simulink model "TypeA_siso180515_export"  (R2016a)
settings: Solver=ode45  StartTime=0.0  StopTime=12.0  RelTol=1e-3
values from neighbouring files (symbols this model uses):
  gain_actIML = 2.1e-7*1.e+6*20/(2^16)/magIM(inddc)*gain_actIML    [TypeA_reconstruction.m]
  gain_actMNL = 5.1e-6*1.e+6*20/(2^16)/magMN(inddc)*gain_actMNL    [TypeA_reconstruction.m]
  gain_actTML = 1.7e-7*1.e+6*20/(2^16)/magTM(inddc)*gain_actTML    [TypeA_reconstruction.m]
  gainBFL = 0    [main.m]
  gainIPL = 0    [main.m]
  sys1 = sys1_exp    [check_exportvsmake.m]    (also in sumcon2mdlconst_typeA.m = sus.ss)
undefined symbols (not defined in the file or in its folder): cMat_BF, cMat_IM, cMat_MN, cMat_TM, gain_actBFGAS, gain_actBFL, gain_actBFP, gain_actBFR, gain_actBFT, gain_actBFV, gain_actBFY, gain_actF0GAS, gain_actF1GAS, gain_actF2GAS, gain_actF3GAS, gain_actIMP, gain_actIMR, gain_actIMT, gain_actIMV, gain_actIMY, gain_actIPL, gain_actIPT, gain_actIPY, gain_actMNP, gain_actMNR, gain_actMNT, gain_actMNV, gain_actMNY, gain_actTMP, gain_actTMY, gainBFGAS, gainBFP, gainBFR, gainBFT, gainBFV, gainBFY, gainF0GAS, gainF1GAS, gainF2GAS, gainF3GAS, gainHieBFP, gainHieBFR, gainHieBFY, gainHieIML, gainHieIMP, gainHieIMY, gainHieIPL, gainHieIPY, gainHieMNL, gainHieMNP, gainHieMNY, gainIML, gainIMP, gainIMR, gainIMT, gainIMV, gainIMY, gainIPT, gainIPY, gainISC_TML ... (+18)
libraries: cstblocks x57
(part 2 of 2)

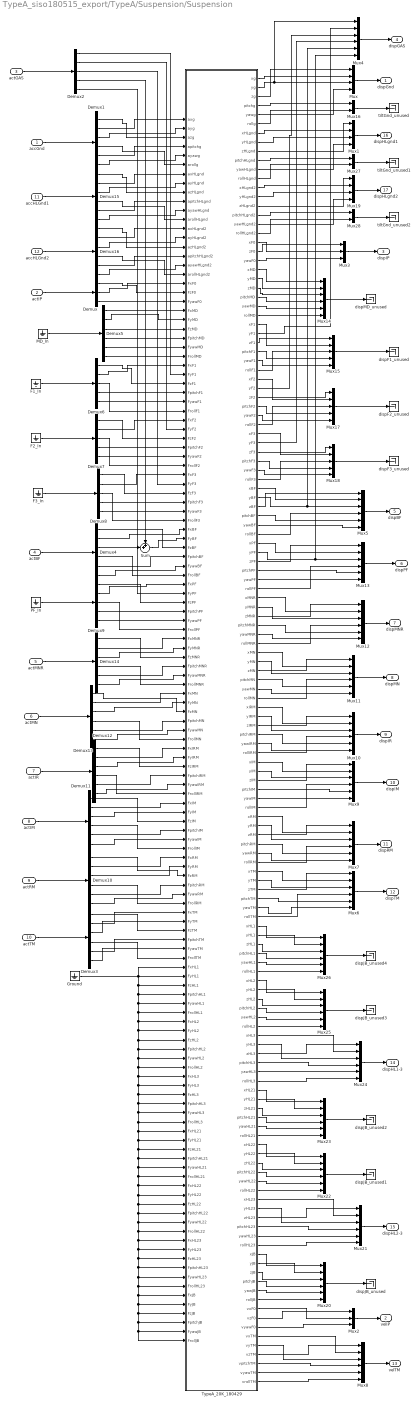
== system TypeA_siso180515_export/TypeA/Suspension/Suspension ==
  accGnd : Inport
  actIP : Inport  Port=2
  actGAS : Inport  Port=3
  actBF : Inport  Port=4
  actMNR : Inport  Port=5
  actMN : Inport  Port=6
  actIR : Inport  Port=7
  actIM : Inport  Port=8
  actRM : Inport  Port=9
  actTM : Inport  Port=10
  accHLGnd1 : Inport  Port=11
  accHLGnd2 : Inport  Port=12
  Demux : Demux  Outputs=3
  Demux{1,3..5,10..16} (11 alike) : Demux  Outputs=6
  Demux{2,6..9} (5 alike) : Demux  Outputs=5
  F1_In : Ground
  F2_In : Ground
  F3_In : Ground
  Ground : Ground
  MD_In : Ground
  Mux : Mux
  Mux1 : Mux
  Mux{4..14,20..26} (18 alike) : Mux  Inputs=6
  Mux15 : Mux  Inputs=5
  Mux16 : Mux  Inputs=2
  Mux17 : Mux  Inputs=5
  Mux18 : Mux  Inputs=5
  Mux19 : Mux
  Mux2 : Mux  Inputs=3
  Mux27 : Mux  Inputs=2
  Mux28 : Mux  Inputs=2
  Mux3 : Mux  Inputs=3
  PF_In : Ground
  Sum : Sum  Inputs=++|
  TypeA_20K_180429 : Subsystem
  dispF1_unused : Terminator
  dispF2_unused : Terminator
  dispF3_unused : Terminator
  dispJB_unused{,1..4} (5 alike) : Terminator
  dispMD_unused : Terminator
  tiltGnd_unused : Terminator
  tiltGnd_unused1 : Terminator
  tiltGnd_unused2 : Terminator
  dispGnd : Outport
  velIP : Outport  Port=2
  dispIP : Outport  Port=3
  dispGAS : Outport  Port=4
  dispBF : Outport  Port=5
  dispPF : Outport  Port=6
  dispMNR : Outport  Port=7
  dispMN : Outport  Port=8
  dispIR : Outport  Port=9
  dispIM : Outport  Port=10
  dispRM : Outport  Port=11
  dispTM : Outport  Port=12
  velTM : Outport  Port=13
  dispHL1-3 : Outport  Port=14
  dispHL2-3 : Outport  Port=15
  dispHLgnd1 : Outport  Port=16
  dispHLgnd2 : Outport  Port=17
  wires:
  Mux/1 -> dispGnd/1
  Mux2/1 -> velIP/1
  Mux3/1 -> dispIP/1
  Mux4/1 -> dispGAS/1
  Mux5/1 -> dispBF/1
  Mux6/1 -> dispTM/1
  actIP/1 -> Demux/1
  accGnd/1 -> Demux1/1
  actTM/1 -> Demux3/1
  Demux4/3 -> Sum/2
  Demux2/4 -> Sum/1
  Demux2/5 -> TypeA_20K_180429/53(FyPF)
  actBF/1 -> Demux4/1
  actGAS/1 -> Demux2/1
  MD_In/1 -> Demux5/1
  Demux5/1 -> TypeA_20K_180429/22(FxMD)
  Demux5/2 -> TypeA_20K_180429/23(FyMD)
  Demux5/3 -> TypeA_20K_180429/24(FzMD)
  Demux5/4 -> TypeA_20K_180429/25(FpitchMD)
  Demux5/5 -> TypeA_20K_180429/26(FyawMD)
  Demux5/6 -> TypeA_20K_180429/27(FrollMD)
  Demux2/1 -> TypeA_20K_180429/29(FyF1)
  Demux2/2 -> TypeA_20K_180429/35(FyF2)
  Demux2/3 -> TypeA_20K_180429/41(FyF3)
  F1_In/1 -> Demux6/1
  F2_In/1 -> Demux7/1
  F3_In/1 -> Demux8/1
  Demux4/1 -> TypeA_20K_180429/48(FzBF)
  PF_In/1 -> Demux9/1
  actRM/1 -> Demux10/1
  actIM/1 -> Demux11/1
  actIR/1 -> Demux12/1
  actMN/1 -> Demux13/1
  actMNR/1 -> Demux14/1
  Demux10/5 -> TypeA_20K_180429/85(FpitchRM)
  Demux10/4 -> TypeA_20K_180429/87(FrollRM)
  Demux10/3 -> TypeA_20K_180429/83(FyRM)
  Demux10/1 -> TypeA_20K_180429/84(FzRM)
  Demux10/2 -> TypeA_20K_180429/82(FxRM)
  Demux3/3 -> TypeA_20K_180429/89(FyTM)
  Demux3/1 -> TypeA_20K_180429/90(FzTM)
  Demux3/2 -> TypeA_20K_180429/88(FxTM)
  Demux3/4 -> TypeA_20K_180429/93(FrollTM)
  Demux3/5 -> TypeA_20K_180429/91(FpitchTM)
  Demux3/6 -> TypeA_20K_180429/92(FyawTM)
  Mux7/1 -> dispRM/1
  Mux8/1 -> velTM/1
  Mux9/1 -> dispIM/1
  Mux10/1 -> dispIR/1
  Mux11/1 -> dispMN/1
  Mux12/1 -> dispMNR/1
  Mux13/1 -> dispPF/1
  Mux14/1 -> dispMD_unused/1
  Mux15/1 -> dispF1_unused/1
  Mux16/1 -> tiltGnd_unused/1
  Mux17/1 -> dispF2_unused/1
  Mux18/1 -> dispF3_unused/1
  TypeA_20K_180429/1(xg) -> Mux/2
  TypeA_20K_180429/3(zg) -> Mux/1
  TypeA_20K_180429/138(vyawF0) -> Mux2/3
  TypeA_20K_180429/19(xF0) -> Mux3/2
  TypeA_20K_180429/20(zF0) -> Mux3/1
  TypeA_20K_180429/21(yawF0) -> Mux3/3
  TypeA_20K_180429/24(zMD) -> Mux14/3
  TypeA_20K_180429/25(pitchMD) -> Mux14/4
  TypeA_20K_180429/26(yawMD) -> Mux14/5
  TypeA_20K_180429/27(rollMD) -> Mux14/6
  TypeA_20K_180429/29(yF1) -> Mux4/2
  TypeA_20K_180429/35(yF2) -> Mux4/3
  TypeA_20K_180429/41(yF3) -> Mux4/4
  TypeA_20K_180429/47(yBF) -> Mux5/3, Mux4/5
  TypeA_20K_180429/53(yPF) -> Mux13/3, Mux4/6
  TypeA_20K_180429/30(zF1) -> Mux15/1
  TypeA_20K_180429/28(xF1) -> Mux15/2
  TypeA_20K_180429/32(yawF1) -> Mux15/5
  TypeA_20K_180429/33(rollF1) -> Mux15/3
  TypeA_20K_180429/31(pitchF1) -> Mux15/4
  TypeA_20K_180429/36(zF2) -> Mux17/1
  TypeA_20K_180429/34(xF2) -> Mux17/2
  TypeA_20K_180429/39(rollF2) -> Mux17/3
  TypeA_20K_180429/38(yawF2) -> Mux17/5
  TypeA_20K_180429/37(pitchF2) -> Mux17/4
  TypeA_20K_180429/42(zF3) -> Mux18/1
  TypeA_20K_180429/40(xF3) -> Mux18/2
  TypeA_20K_180429/44(yawF3) -> Mux18/5
  TypeA_20K_180429/43(pitchF3) -> Mux18/4
  TypeA_20K_180429/45(rollF3) -> Mux18/3
  TypeA_20K_180429/49(pitchBF) -> Mux5/5
  TypeA_20K_180429/50(yawBF) -> Mux5/6
  TypeA_20K_180429/51(rollBF) -> Mux5/4
  TypeA_20K_180429/46(xBF) -> Mux5/2
  TypeA_20K_180429/48(zBF) -> Mux5/1
  TypeA_20K_180429/56(yawPF) -> Mux13/6
  TypeA_20K_180429/54(zPF) -> Mux13/1
  TypeA_20K_180429/52(xPF) -> Mux13/2
  TypeA_20K_180429/57(rollPF) -> Mux13/4
  TypeA_20K_180429/55(pitchPF) -> Mux13/5
  TypeA_20K_180429/58(xMNR) -> Mux12/2
  TypeA_20K_180429/62(yawMNR) -> Mux12/6
  TypeA_20K_180429/59(yMNR) -> Mux12/3
  TypeA_20K_180429/63(rollMNR) -> Mux12/4
  TypeA_20K_180429/60(zMNR) -> Mux12/1
  TypeA_20K_180429/61(pitchMNR) -> Mux12/5
  TypeA_20K_180429/69(rollMN) -> Mux11/4
  TypeA_20K_180429/66(zMN) -> Mux11/1
  TypeA_20K_180429/65(yMN) -> Mux11/3
  TypeA_20K_180429/64(xMN) -> Mux11/2
  TypeA_20K_180429/68(yawMN) -> Mux11/6
  TypeA_20K_180429/67(pitchMN) -> Mux11/5
  TypeA_20K_180429/73(pitchIRM) -> Mux10/5
  TypeA_20K_180429/71(yIRM) -> Mux10/3
  TypeA_20K_180429/74(yawIRM) -> Mux10/6
  TypeA_20K_180429/75(rollIRM) -> Mux10/4
  TypeA_20K_180429/70(xIRM) -> Mux10/2
  TypeA_20K_180429/72(zIRM) -> Mux10/1
  TypeA_20K_180429/78(zIM) -> Mux9/1
  TypeA_20K_180429/77(yIM) -> Mux9/3
  TypeA_20K_180429/76(xIM) -> Mux9/2
  TypeA_20K_180429/141(vzTM) -> Mux8/1
  TypeA_20K_180429/139(vxTM) -> Mux8/2
  TypeA_20K_180429/140(vyTM) -> Mux8/3
  TypeA_20K_180429/142(vpitchTM) -> Mux8/4
  TypeA_20K_180429/143(vyawTM) -> Mux8/5
  TypeA_20K_180429/144(vrollTM) -> Mux8/6
  TypeA_20K_180429/90(zTM) -> Mux6/1
  TypeA_20K_180429/88(xTM) -> Mux6/2
  TypeA_20K_180429/89(yTM) -> Mux6/3
  TypeA_20K_180429/84(zRM) -> Mux7/1
  TypeA_20K_180429/82(xRM) -> Mux7/2
  TypeA_20K_180429/83(yRM) -> Mux7/3
  TypeA_20K_180429/81(rollIM) -> Mux9/4
  TypeA_20K_180429/79(pitchIM) -> Mux9/5
  TypeA_20K_180429/80(yawIM) -> Mux9/6
  TypeA_20K_180429/87(rollRM) -> Mux7/4
  TypeA_20K_180429/85(pitchRM) -> Mux7/5
  TypeA_20K_180429/86(yawRM) -> Mux7/6
  TypeA_20K_180429/93(rollTM) -> Mux6/4
  TypeA_20K_180429/91(pitchTM) -> Mux6/5
  TypeA_20K_180429/92(yawTM) -> Mux6/6
  TypeA_20K_180429/22(xMD) -> Mux14/1
  TypeA_20K_180429/23(yMD) -> Mux14/2
  TypeA_20K_180429/136(vxF0) -> Mux2/2
  TypeA_20K_180429/137(vzF0) -> Mux2/1
  TypeA_20K_180429/2(yg) -> Mux4/1, Mux/3
  TypeA_20K_180429/5(yawg) -> Mux/4
  TypeA_20K_180429/4(pitchg) -> Mux16/1
  TypeA_20K_180429/6(rollg) -> Mux16/2
  Demux10/6 -> TypeA_20K_180429/86(FyawRM)
  Demux11/1 -> TypeA_20K_180429/78(FzIM)
  Demux11/2 -> TypeA_20K_180429/76(FxIM)
  Demux11/3 -> TypeA_20K_180429/77(FyIM)
  Demux11/4 -> TypeA_20K_180429/81(FrollIM)
  Demux11/5 -> TypeA_20K_180429/79(FpitchIM)
  Demux11/6 -> TypeA_20K_180429/80(FyawIM)
  Demux12/1 -> TypeA_20K_180429/72(FzIRM)
  Demux12/2 -> TypeA_20K_180429/70(FxIRM)
  Demux12/3 -> TypeA_20K_180429/71(FyIRM)
  Demux12/4 -> TypeA_20K_180429/75(FrollIRM)
  Demux12/5 -> TypeA_20K_180429/73(FpitchIRM)
  Demux12/6 -> TypeA_20K_180429/74(FyawIRM)
  Demux13/1 -> TypeA_20K_180429/66(FzMN)
  Demux13/2 -> TypeA_20K_180429/64(FxMN)
  Demux13/3 -> TypeA_20K_180429/65(FyMN)
  Demux13/4 -> TypeA_20K_180429/69(FrollMN)
  Demux13/5 -> TypeA_20K_180429/67(FpitchMN)
  Demux13/6 -> TypeA_20K_180429/68(FyawMN)
  Demux14/1 -> TypeA_20K_180429/60(FzMNR)
  Demux14/2 -> TypeA_20K_180429/58(FxMNR)
  Demux14/3 -> TypeA_20K_180429/59(FyMNR)
  Demux14/4 -> TypeA_20K_180429/63(FrollMNR)
  Demux14/5 -> TypeA_20K_180429/61(FpitchMNR)
  Demux14/6 -> TypeA_20K_180429/62(FyawMNR)
  Demux9/1 -> TypeA_20K_180429/54(FzPF)
  Demux9/2 -> TypeA_20K_180429/52(FxPF)
  Demux9/3 -> TypeA_20K_180429/57(FrollPF)
  Demux9/4 -> TypeA_20K_180429/55(FpitchPF)
  Demux9/5 -> TypeA_20K_180429/56(FyawPF)
  Demux4/2 -> TypeA_20K_180429/46(FxBF)
  Sum/1 -> TypeA_20K_180429/47(FyBF)
  Demux4/4 -> TypeA_20K_180429/51(FrollBF)
  Demux4/5 -> TypeA_20K_180429/49(FpitchBF)
  Demux4/6 -> TypeA_20K_180429/50(FyawBF)
  Demux8/1 -> TypeA_20K_180429/42(FzF3)
  Demux8/2 -> TypeA_20K_180429/40(FxF3)
  Demux8/3 -> TypeA_20K_180429/45(FrollF3)
  Demux8/4 -> TypeA_20K_180429/43(FpitchF3)
  Demux8/5 -> TypeA_20K_180429/44(FyawF3)
  Demux7/1 -> TypeA_20K_180429/36(FzF2)
  Demux7/2 -> TypeA_20K_180429/34(FxF2)
  Demux7/3 -> TypeA_20K_180429/39(FrollF2)
  Demux7/4 -> TypeA_20K_180429/37(FpitchF2)
  Demux7/5 -> TypeA_20K_180429/38(FyawF2)
  Demux6/1 -> TypeA_20K_180429/30(FzF1)
  Demux6/2 -> TypeA_20K_180429/28(FxF1)
  Demux6/3 -> TypeA_20K_180429/33(FrollF1)
  Demux6/4 -> TypeA_20K_180429/31(FpitchF1)
  Demux6/5 -> TypeA_20K_180429/32(FyawF1)
  Demux/1 -> TypeA_20K_180429/20(FzF0)
  Demux/2 -> TypeA_20K_180429/19(FxF0)
  Demux/3 -> TypeA_20K_180429/21(FyawF0)
  Demux1/1 -> TypeA_20K_180429/3(azg)
  Demux1/2 -> TypeA_20K_180429/1(axg)
  Demux1/3 -> TypeA_20K_180429/2(ayg)
  Demux1/4 -> TypeA_20K_180429/6(arollg)
  Demux1/5 -> TypeA_20K_180429/4(apitchg)
  Demux1/6 -> TypeA_20K_180429/5(ayawg)
  TypeA_20K_180429/132(zJB) -> Mux20/3
  TypeA_20K_180429/131(yJB) -> Mux20/2
  TypeA_20K_180429/134(yawJB) -> Mux20/5
  TypeA_20K_180429/135(rollJB) -> Mux20/6
  TypeA_20K_180429/130(xJB) -> Mux20/1
  TypeA_20K_180429/133(pitchJB) -> Mux20/4
  Mux20/1 -> dispJB_unused/1
  TypeA_20K_180429/128(yawHL23) -> Mux21/5
  TypeA_20K_180429/129(rollHL23) -> Mux21/6
  TypeA_20K_180429/124(xHL23) -> Mux21/2
  TypeA_20K_180429/127(pitchHL23) -> Mux21/4
  TypeA_20K_180429/125(yHL23) -> Mux21/3
  TypeA_20K_180429/126(zHL23) -> Mux21/1
  Mux21/1 -> dispHL2-3/1
  TypeA_20K_180429/122(yawHL22) -> Mux22/5
  TypeA_20K_180429/120(zHL22) -> Mux22/3
  TypeA_20K_180429/119(yHL22) -> Mux22/2
  TypeA_20K_180429/121(pitchHL22) -> Mux22/4
  TypeA_20K_180429/123(rollHL22) -> Mux22/6
  TypeA_20K_180429/118(xHL22) -> Mux22/1
  Mux22/1 -> dispJB_unused1/1
  TypeA_20K_180429/116(yawHL21) -> Mux23/5
  TypeA_20K_180429/114(zHL21) -> Mux23/3
  TypeA_20K_180429/113(yHL21) -> Mux23/2
  TypeA_20K_180429/115(pitchHL21) -> Mux23/4
  TypeA_20K_180429/117(rollHL21) -> Mux23/6
  TypeA_20K_180429/112(xHL21) -> Mux23/1
  Mux23/1 -> dispJB_unused2/1
  TypeA_20K_180429/110(yawHL3) -> Mux24/5
  TypeA_20K_180429/111(rollHL3) -> Mux24/6
  TypeA_20K_180429/109(pitchHL3) -> Mux24/4
  TypeA_20K_180429/107(yHL3) -> Mux24/3
  TypeA_20K_180429/108(zHL3) -> Mux24/1
  TypeA_20K_180429/106(xHL3) -> Mux24/2
  Mux24/1 -> dispHL1-3/1
  TypeA_20K_180429/104(yawHL2) -> Mux25/5
  Mux25/1 -> dispJB_unused3/1
  TypeA_20K_180429/102(zHL2) -> Mux25/3
  TypeA_20K_180429/103(pitchHL2) -> Mux25/4
  TypeA_20K_180429/105(rollHL2) -> Mux25/6
  TypeA_20K_180429/100(xHL2) -> Mux25/1
  TypeA_20K_180429/101(yHL2) -> Mux25/2
  TypeA_20K_180429/98(yawHL1) -> Mux26/5
  Mux26/1 -> dispJB_unused4/1
  TypeA_20K_180429/96(zHL1) -> Mux26/3
  TypeA_20K_180429/97(pitchHL1) -> Mux26/4
  TypeA_20K_180429/99(rollHL1) -> Mux26/6
  TypeA_20K_180429/94(xHL1) -> Mux26/1
  TypeA_20K_180429/95(yHL1) -> Mux26/2
  TypeA_20K_180429/9(zHLgnd) -> Mux1/1
  TypeA_20K_180429/7(xHLgnd) -> Mux1/2
  TypeA_20K_180429/8(yHLgnd) -> Mux1/3
  TypeA_20K_180429/11(yawHLgnd) -> Mux1/4
  Mux1/1 -> dispHLgnd1/1
  Mux19/1 -> dispHLgnd2/1
  TypeA_20K_180429/14(yHLgnd2) -> Mux19/3
  TypeA_20K_180429/15(zHLgnd2) -> Mux19/1
  TypeA_20K_180429/13(xHLgnd2) -> Mux19/2
  TypeA_20K_180429/17(yawHLgnd2) -> Mux19/4
  TypeA_20K_180429/10(pitchHLgnd) -> Mux27/1
  TypeA_20K_180429/12(rollHLgnd) -> Mux27/2
  Mux27/1 -> tiltGnd_unused1/1
  TypeA_20K_180429/16(pitchHLgnd2) -> Mux28/1
  TypeA_20K_180429/18(rollHLgnd2) -> Mux28/2
  Mux28/1 -> tiltGnd_unused2/1
  Ground/1 -> TypeA_20K_180429/96(FzHL1), TypeA_20K_180429/97(FpitchHL1), TypeA_20K_180429/98(FyawHL1), TypeA_20K_180429/99(FrollHL1), TypeA_20K_180429/100(FxHL2), TypeA_20K_180429/101(FyHL2), TypeA_20K_180429/102(FzHL2), TypeA_20K_180429/103(FpitchHL2), TypeA_20K_180429/104(FyawHL2), TypeA_20K_180429/105(FrollHL2), TypeA_20K_180429/106(FxHL3), TypeA_20K_180429/107(FyHL3), TypeA_20K_180429/108(FzHL3), TypeA_20K_180429/109(FpitchHL3), TypeA_20K_180429/110(FyawHL3), TypeA_20K_180429/111(FrollHL3), TypeA_20K_180429/112(FxHL21), TypeA_20K_180429/113(FyHL21), TypeA_20K_180429/114(FzHL21), TypeA_20K_180429/115(FpitchHL21), TypeA_20K_180429/116(FyawHL21), TypeA_20K_180429/117(FrollHL21), TypeA_20K_180429/118(FxHL22), TypeA_20K_180429/119(FyHL22), TypeA_20K_180429/120(FzHL22), TypeA_20K_180429/121(FpitchHL22), TypeA_20K_180429/122(FyawHL22), TypeA_20K_180429/123(FrollHL22), TypeA_20K_180429/124(FxHL23), TypeA_20K_180429/125(FyHL23), TypeA_20K_180429/126(FzHL23), TypeA_20K_180429/127(FpitchHL23), TypeA_20K_180429/128(FyawHL23), TypeA_20K_180429/129(FrollHL23), TypeA_20K_180429/130(FxJB), TypeA_20K_180429/131(FyJB), TypeA_20K_180429/132(FzJB), TypeA_20K_180429/133(FpitchJB), TypeA_20K_180429/134(FyawJB), TypeA_20K_180429/135(FrollJB), TypeA_20K_180429/95(FyHL1), TypeA_20K_180429/94(FxHL1)
  Demux15/4 -> TypeA_20K_180429/12(arollHLgnd)
  Demux15/5 -> TypeA_20K_180429/10(apitchHLgnd)
  Demux15/1 -> TypeA_20K_180429/9(azHLgnd)
  Demux15/2 -> TypeA_20K_180429/7(axHLgnd)
  Demux15/6 -> TypeA_20K_180429/11(ayawHLgnd)
  accHLGnd1/1 -> Demux15/1
  Demux15/3 -> TypeA_20K_180429/8(ayHLgnd)
  Demux16/4 -> TypeA_20K_180429/18(arollHLgnd2)
  Demux16/5 -> TypeA_20K_180429/16(apitchHLgnd2)
  Demux16/1 -> TypeA_20K_180429/15(azHLgnd2)
  Demux16/2 -> TypeA_20K_180429/13(axHLgnd2)
  Demux16/6 -> TypeA_20K_180429/17(ayawHLgnd2)
  accHLGnd2/1 -> Demux16/1
  Demux16/3 -> TypeA_20K_180429/14(ayHLgnd2)

== system TypeA_siso180515_export/TypeA/Suspension/aMatrix_BF ==
  aMat_in : Inport
  cMat_BF : Constant  Value=cMat_BF  VectorParams1D=off
  coupling_BF : Product  Multiplication=Matrix(*)
  actBF : Outport
  wires:
  coupling_BF/1 -> actBF/1
  aMat_in/1 -> coupling_BF/2
  cMat_BF/1 -> coupling_BF/1

== system TypeA_siso180515_export/TypeA/Suspension/aMatrix_GAS ==
  aMat_in : Inport
  Add{1..4} (4 alike) : Sum  Inputs=+-
  Demux4 : Demux  Outputs=5
  Mux3 : Mux  Inputs=5
  actGAS : Outport
  wires:
  aMat_in/1 -> Demux4/1
  Mux3/1 -> actGAS/1
  Add1/1 -> Mux3/1
  Add2/1 -> Mux3/2
  Demux4/3 -> Add3/1, Add2/2
  Demux4/2 -> Add1/2, Add2/1
  Demux4/1 -> Add1/1
  Demux4/5 -> Mux3/5, Add4/2
  Add4/1 -> Mux3/4
  Add3/1 -> Mux3/3
  Demux4/4 -> Add3/2, Add4/1

== system TypeA_siso180515_export/TypeA/Suspension/aMatrix_IM ==
  aMat_in : Inport
  Gain : Gain  Gain=-1
  cMat_IM : Constant  Value=cMat_IM  VectorParams1D=off
  coupling_IM : Product  Multiplication=Matrix(*)
  actIR : Outport
  actIM : Outport  Port=2
  wires:
  coupling_IM/1 -> actIM/1, Gain/1
  aMat_in/1 -> coupling_IM/2
  cMat_IM/1 -> coupling_IM/1
  Gain/1 -> actIR/1

== system TypeA_siso180515_export/TypeA/Suspension/aMatrix_MN ==
  aMat_in : Inport
  Gain : Gain  Gain=-1
  cMat_MN : Constant  Value=cMat_MN  VectorParams1D=off
  coupling_MN : Product  Multiplication=Matrix(*)
  actMNR : Outport
  actMN : Outport  Port=2
  wires:
  coupling_MN/1 -> actMN/1, Gain/1
  aMat_in/1 -> coupling_MN/2
  cMat_MN/1 -> coupling_MN/1
  Gain/1 -> actMNR/1

== system TypeA_siso180515_export/TypeA/Suspension/aMatrix_TM ==
  aMat_in : Inport
  Demux : Demux  Outputs=3
  Demux1 : Demux  Outputs=3
  Gain : Gain  Gain=-1
  Ground{,1..5} (6 alike) : Ground
  Mux : Mux  Inputs=6
  Mux1 : Mux  Inputs=6
  cMat_TM : Constant  Value=cMat_TM  VectorParams1D=off
  coupling_TM : Product  Multiplication=Matrix(*)
  actRM : Outport
  actTM : Outport  Port=2
  wires:
  coupling_TM/1 -> Demux1/1, Gain/1
  aMat_in/1 -> coupling_TM/2  "3DoF"
  cMat_TM/1 -> coupling_TM/1
  Gain/1 -> Demux/1
  Demux/1 -> Mux/1
  Demux/2 -> Mux/5
  Demux/3 -> Mux/6
  Demux1/1 -> Mux1/1
  Demux1/3 -> Mux1/6
  Demux1/2 -> Mux1/5
  Ground/1 -> Mux/2
  Ground1/1 -> Mux/3
  Ground2/1 -> Mux/4
  Ground4/1 -> Mux1/3
  Ground3/1 -> Mux1/2
  Ground5/1 -> Mux1/4
  Mux/1 -> actRM/1  "6DoF"
  Mux1/1 -> actTM/1  "6DoF"

== system TypeA_siso180515_export/TypeA/Suspension/sMatrix_BF_LVDT ==
  dispGnd : Inport
  dispBF : Inport  Port=2
  Add2 : Sum  Inputs=-+
  Demux : Demux
  Ground : Ground
  Ground1 : Ground
  Mux : Mux  Inputs=6
  BF_LVDT : Outport
  wires:
  Add2/1 -> BF_LVDT/1  "6DoF"
  dispBF/1 -> Add2/2  "6DoF"
  dispGnd/1 -> Demux/1  "4DoF"
  Demux/1 -> Mux/1  "L"
  Demux/2 -> Mux/2  "T"
  Demux/3 -> Mux/3  "V"
  Demux/4 -> Mux/6  "Y"
  Ground/1 -> Mux/4  "R"
  Ground1/1 -> Mux/5  "P"
  Mux/1 -> Add2/1

== system TypeA_siso180515_export/TypeA/Suspension/sMatrix_GAS_LVDT ==
  dispGAS : Inport
  Add{1..5} (5 alike) : Sum  Inputs=-+
  Demux4 : Demux  Outputs=6
  Mux3 : Mux  Inputs=5
  GAS_LVDT : Outport
  wires:
  dispGAS/1 -> Demux4/1
  Demux4/1 -> Add2/1  "VGnd = IPV"
  Demux4/2 -> Add1/1, Add2/2  "VF1"
  Demux4/3 -> Add1/2, Add3/1  "VF2"
  Demux4/4 -> Add4/1, Add3/2  "VF3"
  Add2/1 -> Mux3/1  "GASF0"
  Add1/1 -> Mux3/2  "GASF1"
  Add3/1 -> Mux3/3  "GASF2"
  Mux3/1 -> GAS_LVDT/1
  Demux4/5 -> Add5/1, Add4/2  "VBF"
  Demux4/6 -> Add5/2  "VPF"
  Add4/1 -> Mux3/4  "GASF3"
  Add5/1 -> Mux3/5  "GASBF"

== system TypeA_siso180515_export/TypeA/Suspension/sMatrix_IM_PS ==
  dispIR : Inport
  dispIM : Inport  Port=2
  Add2 : Sum  Inputs=-+
  IM_PS : Outport
  wires:
  Add2/1 -> IM_PS/1
  dispIM/1 -> Add2/2
  dispIR/1 -> Add2/1

== system TypeA_siso180515_export/TypeA/Suspension/sMatrix_IP_LVDT ==
  dispGnd : Inport
  dispIP : Inport  Port=2
  Add2 : Sum  Inputs=-+
  Demux : Demux
  Mux : Mux  Inputs=3
  Terminator : Terminator
  IP_LVDT : Outport
  wires:
  Add2/1 -> IP_LVDT/1
  dispIP/1 -> Add2/2
  dispGnd/1 -> Demux/1
  Demux/1 -> Mux/1  "L"
  Demux/2 -> Mux/2  "T"
  Demux/4 -> Mux/3  "Y"
  Demux/3 -> Terminator/1  "V"
  Mux/1 -> Add2/1

== system TypeA_siso180515_export/TypeA/Suspension/sMatrix_MN_OpLev ==
  dispMN : Inport
  Demux4 : Demux  Outputs=6
  Mux3 : Mux  Inputs=3
  dispMNL : Terminator
  dispMNT : Terminator
  dispMNV : Terminator
  MN_OpLev : Outport
  wires:
  dispMN/1 -> Demux4/1
  Mux3/1 -> MN_OpLev/1
  Demux4/1 -> dispMNL/1
  Demux4/2 -> dispMNT/1
  Demux4/3 -> dispMNV/1
  Demux4/4 -> Mux3/1
  Demux4/5 -> Mux3/2
  Demux4/6 -> Mux3/3

== system TypeA_siso180515_export/TypeA/Suspension/sMatrix_MN_PS ==
  dispMNR : Inport
  dispMN : Inport  Port=2
  Add2 : Sum  Inputs=-+
  MN_PS : Outport
  wires:
  Add2/1 -> MN_PS/1
  dispMN/1 -> Add2/2
  dispMNR/1 -> Add2/1

== system TypeA_siso180515_export/TypeA/Suspension/sMatrix_PF_OpLev ==
  dispPF : Inport
  Demux4 : Demux  Outputs=6
  Mux3 : Mux  Inputs=3
  dispLPF : Terminator
  dispTPF : Terminator
  dispVPF : Terminator
  OpLev_PF : Outport
  wires:
  dispPF/1 -> Demux4/1
  Mux3/1 -> OpLev_PF/1
  Demux4/1 -> dispLPF/1
  Demux4/2 -> dispTPF/1
  Demux4/3 -> dispVPF/1
  Demux4/4 -> Mux3/1
  Demux4/5 -> Mux3/2
  Demux4/6 -> Mux3/3

== system TypeA_siso180515_export/TypeA/Suspension/sMatrix_TM_OpLev ==
  dispTM : Inport
  Demux4 : Demux  Outputs=6
  Mux3 : Mux  Inputs=3
  dispTMR : Terminator
  dispTMT : Terminator
  dispTMV : Terminator
  TM_OpLev : Outport
  wires:
  dispTM/1 -> Demux4/1
  Mux3/1 -> TM_OpLev/1
  Demux4/1 -> Mux3/1
  Demux4/2 -> dispTMT/1
  Demux4/3 -> dispTMV/1
  Demux4/4 -> dispTMR/1
  Demux4/5 -> Mux3/2
  Demux4/6 -> Mux3/3

== system TypeA_siso180515_export/TypeA/Suspension/sMatrix_TM_PS ==
  dispRM : Inport
  dispTM : Inport  Port=2
  Add2 : Sum  Inputs=-+
  Demux : Demux  Outputs=6
  Demux1 : Demux  Outputs=6
  Mux : Mux  Inputs=3
  Mux1 : Mux  Inputs=3
  Terminator{,1..5} (6 alike) : Terminator
  TM_PS : Outport
  wires:
  Add2/1 -> TM_PS/1  "(L, P, Y)"
  dispRM/1 -> Demux/1
  dispTM/1 -> Demux1/1
  Demux/1 -> Mux/1  "L"
  Demux/5 -> Mux/2  "P"
  Demux/6 -> Mux/3  "Y"
  Demux1/1 -> Mux1/1  "L"
  Demux1/5 -> Mux1/2  "P"
  Demux1/6 -> Mux1/3  "Y"
  Mux/1 -> Add2/1
  Mux1/1 -> Add2/2
  Demux/2 -> Terminator/1  "T"
  Demux/4 -> Terminator2/1  "R"
  Demux/3 -> Terminator1/1  "V"
  Demux1/4 -> Terminator5/1  "R"
  Demux1/2 -> Terminator3/1  "T"
  Demux1/3 -> Terminator4/1  "V"

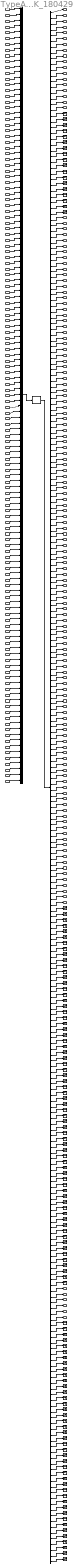
== system TypeA_siso180515_export/TypeA/Suspension/Suspension/TypeA_20K_180429 ==
  axg : Inport
  ayg : Inport  Port=2
  azg : Inport  Port=3
  apitchg : Inport  Port=4
  ayawg : Inport  Port=5
  arollg : Inport  Port=6
  axHLgnd : Inport  Port=7
  ayHLgnd : Inport  Port=8
  azHLgnd : Inport  Port=9
  apitchHLgnd : Inport  Port=10
  ayawHLgnd : Inport  Port=11
  arollHLgnd : Inport  Port=12
  axHLgnd2 : Inport  Port=13
  ayHLgnd2 : Inport  Port=14
  azHLgnd2 : Inport  Port=15
  apitchHLgnd2 : Inport  Port=16
  ayawHLgnd2 : Inport  Port=17
  arollHLgnd2 : Inport  Port=18
  FxF0 : Inport  Port=19
  FzF0 : Inport  Port=20
  FyawF0 : Inport  Port=21
  FxMD : Inport  Port=22
  FyMD : Inport  Port=23
  FzMD : Inport  Port=24
  FpitchMD : Inport  Port=25
  FyawMD : Inport  Port=26
  FrollMD : Inport  Port=27
  FxF1 : Inport  Port=28
  FyF1 : Inport  Port=29
  FzF1 : Inport  Port=30
  FpitchF1 : Inport  Port=31
  FyawF1 : Inport  Port=32
  FrollF1 : Inport  Port=33
  FxF2 : Inport  Port=34
  FyF2 : Inport  Port=35
  FzF2 : Inport  Port=36
  FpitchF2 : Inport  Port=37
  FyawF2 : Inport  Port=38
  FrollF2 : Inport  Port=39
  FxF3 : Inport  Port=40
  FyF3 : Inport  Port=41
  FzF3 : Inport  Port=42
  FpitchF3 : Inport  Port=43
  FyawF3 : Inport  Port=44
  FrollF3 : Inport  Port=45
  FxBF : Inport  Port=46
  FyBF : Inport  Port=47
  FzBF : Inport  Port=48
  FpitchBF : Inport  Port=49
  FyawBF : Inport  Port=50
  FrollBF : Inport  Port=51
  FxPF : Inport  Port=52
  FyPF : Inport  Port=53
  FzPF : Inport  Port=54
  FpitchPF : Inport  Port=55
  FyawPF : Inport  Port=56
  FrollPF : Inport  Port=57
  FxMNR : Inport  Port=58
  FyMNR : Inport  Port=59
  FzMNR : Inport  Port=60
  FpitchMNR : Inport  Port=61
  FyawMNR : Inport  Port=62
  FrollMNR : Inport  Port=63
  FxMN : Inport  Port=64
  FyMN : Inport  Port=65
  FzMN : Inport  Port=66
  FpitchMN : Inport  Port=67
  FyawMN : Inport  Port=68
  FrollMN : Inport  Port=69
  FxIRM : Inport  Port=70
  FyIRM : Inport  Port=71
  FzIRM : Inport  Port=72
  FpitchIRM : Inport  Port=73
  FyawIRM : Inport  Port=74
  FrollIRM : Inport  Port=75
  FxIM : Inport  Port=76
  FyIM : Inport  Port=77
  FzIM : Inport  Port=78
  FpitchIM : Inport  Port=79
  FyawIM : Inport  Port=80
  FrollIM : Inport  Port=81
  FxRM : Inport  Port=82
  FyRM : Inport  Port=83
  FzRM : Inport  Port=84
  FpitchRM : Inport  Port=85
  FyawRM : Inport  Port=86
  FrollRM : Inport  Port=87
  FxTM : Inport  Port=88
  FyTM : Inport  Port=89
  FzTM : Inport  Port=90
  FpitchTM : Inport  Port=91
  FyawTM : Inport  Port=92
  FrollTM : Inport  Port=93
  FxHL1 : Inport  Port=94
  FyHL1 : Inport  Port=95
  FzHL1 : Inport  Port=96
  FpitchHL1 : Inport  Port=97
  FyawHL1 : Inport  Port=98
  FrollHL1 : Inport  Port=99
  FxHL2 : Inport  Port=100
  FyHL2 : Inport  Port=101
  FzHL2 : Inport  Port=102
  FpitchHL2 : Inport  Port=103
  FyawHL2 : Inport  Port=104
  FrollHL2 : Inport  Port=105
  FxHL3 : Inport  Port=106
  FyHL3 : Inport  Port=107
  FzHL3 : Inport  Port=108
  FpitchHL3 : Inport  Port=109
  FyawHL3 : Inport  Port=110
  FrollHL3 : Inport  Port=111
  FxHL21 : Inport  Port=112
  FyHL21 : Inport  Port=113
  FzHL21 : Inport  Port=114
  FpitchHL21 : Inport  Port=115
  FyawHL21 : Inport  Port=116
  FrollHL21 : Inport  Port=117
  FxHL22 : Inport  Port=118
  FyHL22 : Inport  Port=119
  FzHL22 : Inport  Port=120
  FpitchHL22 : Inport  Port=121
  FyawHL22 : Inport  Port=122
  FrollHL22 : Inport  Port=123
  FxHL23 : Inport  Port=124
  FyHL23 : Inport  Port=125
  FzHL23 : Inport  Port=126
  FpitchHL23 : Inport  Port=127
  FyawHL23 : Inport  Port=128
  FrollHL23 : Inport  Port=129
  FxJB : Inport  Port=130
  FyJB : Inport  Port=131
  FzJB : Inport  Port=132
  FpitchJB : Inport  Port=133
  FyawJB : Inport  Port=134
  FrollJB : Inport  Port=135
  SAS State-Space : StateSpace  A=sys1.A  B=sys1.B  C=sys1.C  D=sys1.D  X0=0  ContinuousStateAttributes='SUS_SS_MODEL'
  Terminator{,1..125} (126 alike) : Terminator
  demux : Demux  Outputs=270
  mux : Mux  Inputs=135
  xg : Outport
  yg : Outport  Port=2
  zg : Outport  Port=3
  pitchg : Outport  Port=4
  yawg : Outport  Port=5
  rollg : Outport  Port=6
  xHLgnd : Outport  Port=7
  yHLgnd : Outport  Port=8
  zHLgnd : Outport  Port=9
  pitchHLgnd : Outport  Port=10
  yawHLgnd : Outport  Port=11
  rollHLgnd : Outport  Port=12
  xHLgnd2 : Outport  Port=13
  yHLgnd2 : Outport  Port=14
  zHLgnd2 : Outport  Port=15
  pitchHLgnd2 : Outport  Port=16
  yawHLgnd2 : Outport  Port=17
  rollHLgnd2 : Outport  Port=18
  xF0 : Outport  Port=19
  zF0 : Outport  Port=20
  yawF0 : Outport  Port=21
  xMD : Outport  Port=22
  yMD : Outport  Port=23
  zMD : Outport  Port=24
  pitchMD : Outport  Port=25
  yawMD : Outport  Port=26
  rollMD : Outport  Port=27
  xF1 : Outport  Port=28
  yF1 : Outport  Port=29
  zF1 : Outport  Port=30
  pitchF1 : Outport  Port=31
  yawF1 : Outport  Port=32
  rollF1 : Outport  Port=33
  xF2 : Outport  Port=34
  yF2 : Outport  Port=35
  zF2 : Outport  Port=36
  pitchF2 : Outport  Port=37
  yawF2 : Outport  Port=38
  rollF2 : Outport  Port=39
  xF3 : Outport  Port=40
  yF3 : Outport  Port=41
  zF3 : Outport  Port=42
  pitchF3 : Outport  Port=43
  yawF3 : Outport  Port=44
  rollF3 : Outport  Port=45
  xBF : Outport  Port=46
  yBF : Outport  Port=47
  zBF : Outport  Port=48
  pitchBF : Outport  Port=49
  yawBF : Outport  Port=50
  rollBF : Outport  Port=51
  xPF : Outport  Port=52
  yPF : Outport  Port=53
  zPF : Outport  Port=54
  pitchPF : Outport  Port=55
  yawPF : Outport  Port=56
  rollPF : Outport  Port=57
  xMNR : Outport  Port=58
  yMNR : Outport  Port=59
  zMNR : Outport  Port=60
  pitchMNR : Outport  Port=61
  yawMNR : Outport  Port=62
  rollMNR : Outport  Port=63
  xMN : Outport  Port=64
  yMN : Outport  Port=65
  zMN : Outport  Port=66
  pitchMN : Outport  Port=67
  yawMN : Outport  Port=68
  rollMN : Outport  Port=69
  xIRM : Outport  Port=70
  yIRM : Outport  Port=71
  zIRM : Outport  Port=72
  pitchIRM : Outport  Port=73
  yawIRM : Outport  Port=74
  rollIRM : Outport  Port=75
  xIM : Outport  Port=76
  yIM : Outport  Port=77
  zIM : Outport  Port=78
  pitchIM : Outport  Port=79
  yawIM : Outport  Port=80
  rollIM : Outport  Port=81
  xRM : Outport  Port=82
  yRM : Outport  Port=83
  zRM : Outport  Port=84
  pitchRM : Outport  Port=85
  yawRM : Outport  Port=86
  rollRM : Outport  Port=87
  xTM : Outport  Port=88
  yTM : Outport  Port=89
  zTM : Outport  Port=90
  pitchTM : Outport  Port=91
  yawTM : Outport  Port=92
  rollTM : Outport  Port=93
  xHL1 : Outport  Port=94
  yHL1 : Outport  Port=95
  zHL1 : Outport  Port=96
  pitchHL1 : Outport  Port=97
  yawHL1 : Outport  Port=98
  rollHL1 : Outport  Port=99
  xHL2 : Outport  Port=100
  yHL2 : Outport  Port=101
  zHL2 : Outport  Port=102
  pitchHL2 : Outport  Port=103
  yawHL2 : Outport  Port=104
  rollHL2 : Outport  Port=105
  xHL3 : Outport  Port=106
  yHL3 : Outport  Port=107
  zHL3 : Outport  Port=108
  pitchHL3 : Outport  Port=109
  yawHL3 : Outport  Port=110
  rollHL3 : Outport  Port=111
  xHL21 : Outport  Port=112
  yHL21 : Outport  Port=113
  zHL21 : Outport  Port=114
  pitchHL21 : Outport  Port=115
  yawHL21 : Outport  Port=116
  rollHL21 : Outport  Port=117
  xHL22 : Outport  Port=118
  yHL22 : Outport  Port=119
  zHL22 : Outport  Port=120
  pitchHL22 : Outport  Port=121
  yawHL22 : Outport  Port=122
  rollHL22 : Outport  Port=123
  xHL23 : Outport  Port=124
  yHL23 : Outport  Port=125
  zHL23 : Outport  Port=126
  pitchHL23 : Outport  Port=127
  yawHL23 : Outport  Port=128
  rollHL23 : Outport  Port=129
  xJB : Outport  Port=130
  yJB : Outport  Port=131
  zJB : Outport  Port=132
  pitchJB : Outport  Port=133
  yawJB : Outport  Port=134
  rollJB : Outport  Port=135
  vxF0 : Outport  Port=136
  vzF0 : Outport  Port=137
  vyawF0 : Outport  Port=138
  vxTM : Outport  Port=139
  vyTM : Outport  Port=140
  vzTM : Outport  Port=141
  vpitchTM : Outport  Port=142
  vyawTM : Outport  Port=143
  vrollTM : Outport  Port=144
  wires:
  demux/165 -> Terminator26/1
  demux/265 -> Terminator120/1
  demux/247 -> Terminator102/1
  demux/191 -> Terminator52/1
  FrollHL23/1 -> mux/129
  demux/163 -> Terminator24/1
  FzIM/1 -> mux/78
  demux/263 -> Terminator118/1
  demux/260 -> Terminator115/1
  SAS State-Space/1 -> demux/1
  arollHLgnd2/1 -> mux/18
  demux/236 -> Terminator91/1
  demux/256 -> Terminator111/1
  demux/183 -> Terminator44/1
  demux/255 -> Terminator110/1
  demux/242 -> Terminator97/1
  demux/252 -> Terminator107/1
  demux/137 -> yHL22/1
  demux/75 -> rollPF/1
  demux/234 -> Terminator89/1
  FzF1/1 -> mux/30
  demux/177 -> Terminator38/1
  FzF3/1 -> mux/42
  demux/251 -> Terminator106/1
  demux/243 -> Terminator98/1
  demux/227 -> vyawTM/1
  demux/173 -> Terminator34/1
  demux/78 -> zMNR/1
  demux/106 -> xTM/1
  demux/228 -> vrollTM/1
  demux/246 -> Terminator101/1
  demux/120 -> zHL2/1
  demux/223 -> vxTM/1
  demux/239 -> Terminator94/1
  demux/241 -> Terminator96/1
  demux/216 -> Terminator77/1
  demux/215 -> Terminator76/1
  demux/107 -> yTM/1
  demux/206 -> Terminator67/1
  demux/235 -> Terminator90/1
  demux/237 -> Terminator92/1
  demux/203 -> Terminator64/1
  demux/233 -> Terminator88/1
  demux/224 -> vyTM/1
  demux/155 -> vzF0/1
  demux/266 -> Terminator121/1
  demux/238 -> Terminator93/1
  demux/270 -> Terminator125/1
  demux/232 -> Terminator87/1
  demux/244 -> Terminator99/1
  FzIRM/1 -> mux/72
  demux/248 -> Terminator103/1
  FyF3/1 -> mux/41
  demux/253 -> Terminator108/1
  demux/249 -> Terminator104/1
  demux/122 -> yawHL2/1
  demux/175 -> Terminator36/1
  demux/202 -> Terminator63/1
  demux/268 -> Terminator123/1
  demux/164 -> Terminator25/1
  demux/218 -> Terminator79/1
  FzHL1/1 -> mux/96
  demux/261 -> Terminator116/1
  demux/254 -> Terminator109/1
  demux/269 -> Terminator124/1
  demux/174 -> Terminator35/1
  demux/57 -> rollF2/1
  demux/171 -> Terminator32/1
  FyBF/1 -> mux/47
  FyawIM/1 -> mux/80
  demux/176 -> Terminator37/1
  FpitchMNR/1 -> mux/61
  demux/140 -> yawHL22/1
  demux/149 -> yJB/1
  demux/146 -> yawHL23/1
  demux/226 -> vpitchTM/1
  demux/162 -> Terminator23/1
  FxMNR/1 -> mux/58
  demux/74 -> yawPF/1
  demux/56 -> yawF2/1
  demux/153 -> rollJB/1
  demux/219 -> Terminator80/1
  FrollTM/1 -> mux/93
  demux/142 -> xHL23/1
  demux/240 -> Terminator95/1
  demux/159 -> Terminator20/1
  demux/145 -> pitchHL23/1
  demux/130 -> xHL21/1
  demux/204 -> Terminator65/1
  demux/129 -> rollHL3/1
  demux/128 -> yawHL3/1
  FpitchMD/1 -> mux/25
  demux/135 -> rollHL21/1
  axg/1 -> mux/1
  demux/267 -> Terminator122/1
  demux/139 -> pitchHL22/1
  demux/136 -> xHL22/1
  demux/222 -> Terminator83/1
  demux/131 -> yHL21/1
  demux/73 -> pitchPF/1
  demux/121 -> pitchHL2/1
  demux/104 -> yawRM/1
  apitchg/1 -> mux/4
  demux/250 -> Terminator105/1
  demux/124 -> xHL3/1
  demux/113 -> yHL1/1
  demux/117 -> rollHL1/1
  demux/63 -> rollF3/1
  demux/109 -> pitchTM/1
  demux/126 -> zHL3/1
  demux/198 -> Terminator59/1
  demux/96 -> zIM/1
  FzMD/1 -> mux/24
  demux/264 -> Terminator119/1
  FrollMD/1 -> mux/27
  FzHL21/1 -> mux/114
  demux/112 -> xHL1/1
  demux/144 -> zHL23/1
  FxF1/1 -> mux/28
  demux/108 -> zTM/1
  demux/213 -> Terminator74/1
  demux/102 -> zRM/1
  FyawF1/1 -> mux/32
  demux/211 -> Terminator72/1
  demux/94 -> xIM/1
  demux/41 -> yMD/1
  demux/101 -> yRM/1
  demux/158 -> Terminator19/1
  demux/103 -> pitchRM/1
  demux/152 -> yawJB/1
  demux/231 -> Terminator86/1
  demux/15 -> zHLgnd2/1
  demux/46 -> xF1/1
  demux/127 -> pitchHL3/1
  demux/38 -> zF0/1
  FxMD/1 -> mux/22
  demux/86 -> yawMN/1
  demux/91 -> pitchIRM/1
  FyawRM/1 -> mux/86
  demux/262 -> Terminator117/1
  demux/89 -> yIRM/1
  demux/8 -> yHLgnd/1
  demux/81 -> rollMNR/1
  demux/123 -> rollHL2/1
  demux/19 -> Terminator/1
  demux/168 -> Terminator29/1
  demux/77 -> yMNR/1
  demux/80 -> yawMNR/1
  demux/79 -> pitchMNR/1
  demux/58 -> xF3/1
  demux/82 -> xMN/1
  demux/210 -> Terminator71/1
  demux/68 -> yawBF/1
  demux/54 -> zF2/1
  demux/26 -> Terminator7/1
  demux/66 -> zBF/1
  demux/64 -> xBF/1
  demux/125 -> yHL3/1
  FyRM/1 -> mux/83
  FyPF/1 -> mux/53
  demux/53 -> yF2/1
  FyHL1/1 -> mux/95
  demux/225 -> vzTM/1
  demux/60 -> zF3/1
  demux/220 -> Terminator81/1
  demux/199 -> Terminator60/1
  FxF0/1 -> mux/19
  FzF2/1 -> mux/36
  demux/52 -> xF2/1
  FrollHL3/1 -> mux/111
  demux/43 -> pitchMD/1
  demux/22 -> Terminator3/1
  demux/92 -> yawIRM/1
  demux/150 -> zJB/1
  demux/13 -> xHLgnd2/1
  demux/40 -> xMD/1
  demux/50 -> yawF1/1
  demux/49 -> pitchF1/1
  demux/118 -> xHL2/1
  demux/99 -> rollIM/1
  demux/44 -> yawMD/1
  demux/48 -> zF1/1
  demux/134 -> yawHL21/1
  FxPF/1 -> mux/52
  demux/28 -> Terminator9/1
  demux/62 -> yawF3/1
  demux/132 -> zHL21/1
  demux/4 -> pitchg/1
  FyF1/1 -> mux/29
  FyJB/1 -> mux/131
  FrollHL22/1 -> mux/123
  demux/100 -> xRM/1
  demux/2 -> yg/1
  demux/105 -> rollRM/1
  demux/5 -> yawg/1
  demux/72 -> zPF/1
  demux/115 -> pitchHL1/1
  demux/3 -> zg/1
  FyawMD/1 -> mux/26
  FzJB/1 -> mux/132
  demux/110 -> yawTM/1
  FrollIM/1 -> mux/81
  FrollJB/1 -> mux/135
  demux/6 -> rollg/1
  demux/67 -> pitchBF/1
  FzHL23/1 -> mux/126
  demux/160 -> Terminator21/1
  FzHL3/1 -> mux/108
  FpitchHL22/1 -> mux/121
  FpitchHL21/1 -> mux/115
  demux/70 -> xPF/1
  FrollHL21/1 -> mux/117
  FyawHL22/1 -> mux/122
  FxJB/1 -> mux/130
  demux/85 -> pitchMN/1
  FxHL22/1 -> mux/118
  FxHL23/1 -> mux/124
  FpitchHL2/1 -> mux/103
  FyHL2/1 -> mux/101
  FxHL1/1 -> mux/94
  FpitchHL3/1 -> mux/109
  FyHL21/1 -> mux/113
  demux/65 -> yBF/1
  demux/116 -> yawHL1/1
  FyawHL2/1 -> mux/104
  FxTM/1 -> mux/88
  FyHL3/1 -> mux/107
  FxHL3/1 -> mux/106
  FyawTM/1 -> mux/92
  FyawF2/1 -> mux/38
  demux/258 -> Terminator113/1
  FzHL2/1 -> mux/102
  FpitchTM/1 -> mux/91
  FyawHL3/1 -> mux/110
  FyawHL21/1 -> mux/116
  FyawHL1/1 -> mux/98
  FrollHL2/1 -> mux/105
  demux/24 -> Terminator5/1
  FrollHL1/1 -> mux/99
  demux/133 -> pitchHL21/1
  demux/178 -> Terminator39/1
  FyawIRM/1 -> mux/74
  demux/166 -> Terminator27/1
  FxIRM/1 -> mux/70
  FpitchRM/1 -> mux/85
  FyawMNR/1 -> mux/62
  demux/257 -> Terminator112/1
  FrollMNR/1 -> mux/63
  FpitchHL23/1 -> mux/127
  FyMN/1 -> mux/65
  FxRM/1 -> mux/82
  demux/51 -> rollF1/1
  demux/7 -> xHLgnd/1
  FrollMN/1 -> mux/69
  FpitchIM/1 -> mux/79
  demux/27 -> Terminator8/1
  FxMN/1 -> mux/64
  FzHL22/1 -> mux/120
  FzMN/1 -> mux/66
  FyIRM/1 -> mux/71
  demux/14 -> yHLgnd2/1
  FzMNR/1 -> mux/60
  FzBF/1 -> mux/48
  FrollIRM/1 -> mux/75
  demux/11 -> yawHLgnd/1
  demux/45 -> rollMD/1
  FzF0/1 -> mux/20
  FxHL2/1 -> mux/100
  FyawPF/1 -> mux/56
  demux/10 -> pitchHLgnd/1
  demux/20 -> Terminator1/1
  FpitchPF/1 -> mux/55
  demux/1 -> xg/1
  FrollF1/1 -> mux/33
  FrollF3/1 -> mux/45
  FxHL21/1 -> mux/112
  FzPF/1 -> mux/54
  demux/93 -> rollIRM/1
  FpitchBF/1 -> mux/49
  FyawF3/1 -> mux/44
  FxBF/1 -> mux/46
  FyawF0/1 -> mux/21
  FpitchF3/1 -> mux/43
  demux/47 -> yF1/1
  demux/119 -> yHL2/1
  demux/59 -> yF3/1
  FpitchF2/1 -> mux/37
  FyF2/1 -> mux/35
  apitchHLgnd2/1 -> mux/16
  azHLgnd2/1 -> mux/15
  ayHLgnd2/1 -> mux/14
  FxF2/1 -> mux/34
  arollHLgnd/1 -> mux/12
  FrollPF/1 -> mux/57
  FpitchF1/1 -> mux/31
  axHLgnd/1 -> mux/7
  FzRM/1 -> mux/84
  FxIM/1 -> mux/76
  ayawHLgnd/1 -> mux/11
  demux/230 -> Terminator85/1
  azHLgnd/1 -> mux/9
  ayawg/1 -> mux/5
  azg/1 -> mux/3
  demux/209 -> Terminator70/1
  demux/172 -> Terminator33/1
  demux/259 -> Terminator114/1
  demux/208 -> Terminator69/1
  demux/182 -> Terminator43/1
  FyMD/1 -> mux/23
  demux/200 -> Terminator61/1
  demux/207 -> Terminator68/1
  demux/151 -> pitchJB/1
  demux/201 -> Terminator62/1
  mux/1 -> SAS State-Space/1
  demux/205 -> Terminator66/1
  demux/114 -> zHL1/1
  demux/25 -> Terminator6/1
  demux/197 -> Terminator58/1
  FyawJB/1 -> mux/134
  demux/212 -> Terminator73/1
  demux/214 -> Terminator75/1
  demux/23 -> Terminator4/1
  demux/88 -> xIRM/1
  FpitchHL1/1 -> mux/97
  FrollF2/1 -> mux/39
  demux/188 -> Terminator49/1
  demux/111 -> rollTM/1
  demux/192 -> Terminator53/1
  demux/84 -> zMN/1
  demux/148 -> xJB/1
  demux/179 -> Terminator40/1
  demux/154 -> vxF0/1
  demux/87 -> rollMN/1
  demux/185 -> Terminator46/1
  demux/147 -> rollHL23/1
  demux/167 -> Terminator28/1
  demux/186 -> Terminator47/1
  demux/143 -> yHL23/1
  apitchHLgnd/1 -> mux/10
  ayawHLgnd2/1 -> mux/17
  FzTM/1 -> mux/90
  ayHLgnd/1 -> mux/8
  demux/21 -> Terminator2/1
  FrollRM/1 -> mux/87
  demux/61 -> pitchF3/1
  demux/55 -> pitchF2/1
  demux/83 -> yMN/1
  demux/16 -> pitchHLgnd2/1
  demux/18 -> rollHLgnd2/1
  arollg/1 -> mux/6
  ayg/1 -> mux/2
  demux/98 -> yawIM/1
  FrollBF/1 -> mux/51
  demux/97 -> pitchIM/1
  demux/195 -> Terminator56/1
  FyawBF/1 -> mux/50
  axHLgnd2/1 -> mux/13
  demux/187 -> Terminator48/1
  demux/189 -> Terminator50/1
  demux/221 -> Terminator82/1
  demux/181 -> Terminator42/1
  FyHL22/1 -> mux/119
  demux/156 -> vyawF0/1
  FyIM/1 -> mux/77
  demux/245 -> Terminator100/1
  FyMNR/1 -> mux/59
  demux/170 -> Terminator31/1
  demux/169 -> Terminator30/1
  demux/229 -> Terminator84/1
  FpitchIRM/1 -> mux/73
  demux/194 -> Terminator55/1
  demux/157 -> Terminator18/1
  demux/17 -> yawHLgnd2/1
  demux/42 -> zMD/1
  demux/196 -> Terminator57/1
  demux/180 -> Terminator41/1
  demux/90 -> zIRM/1
  demux/69 -> rollBF/1
  demux/71 -> yPF/1
  demux/39 -> yawF0/1
  FyHL23/1 -> mux/125
  FpitchMN/1 -> mux/67
  FxF3/1 -> mux/40
  demux/76 -> xMNR/1
  demux/193 -> Terminator54/1
  demux/37 -> xF0/1
  FyawMN/1 -> mux/68
  demux/190 -> Terminator51/1
  demux/138 -> zHL22/1
  demux/9 -> zHLgnd/1
  demux/184 -> Terminator45/1
  demux/161 -> Terminator22/1
  demux/217 -> Terminator78/1
  FpitchJB/1 -> mux/133
  demux/141 -> rollHL22/1
  FyawHL23/1 -> mux/128
  demux/95 -> yIM/1
  demux/12 -> rollHLgnd/1
  FyTM/1 -> mux/89
  demux/29 -> Terminator10/1
  demux/30 -> Terminator11/1
  demux/36 -> Terminator12/1
  demux/35 -> Terminator13/1
  demux/34 -> Terminator14/1
  demux/33 -> Terminator15/1
  demux/32 -> Terminator16/1
  demux/31 -> Terminator17/1
